simulink model "Test_PWM"  (R2014a)
settings: Solver=FixedStepDiscrete  StartTime=0.0  StopTime=10.0  FixedStep=0.1  RelTol=1e-3
libraries: GPIO_Lib x2, STM32_Config_Lib x1, TIMERS_Lib x1
settings Model: Creator=jan  LastModifiedBy=jan
settings DataIOCC: LimitDataPoints=off
settings OptimizationCC: OptimizeModelRefInitCode=on  LifeSpan=1
settings HardwareCC: ProdLargestAtomicInteger=Integer  ProdLargestAtomicFloat=Float  ProdIntDivRoundTo=Zero  ProdEndianess=LittleEndian  ProdHWDeviceType=STMicroelectronics->STM32 32-bit Cortex-M
settings RTWCC: SystemTargetFile=stm32.tlc  TemplateMakefile=stm32.tmf  Description=stm32 (Embedded Target)  GenerateReport=on  ProcessScript=stm32_make_rtw_hook  Toolchain=Microsoft Visual C++ 2012 v11.0 | nmake (64-bit Windows)
settings CodeAppCC: IgnoreCustomStorageClasses=off  MaxIdLength=64  CustomSymbolStrType=$N$R$M  SimulinkBlockComments=off
settings STFCustomTargetCC: CodeReplacementLibrary=ARM CMSIS SIN COS  ParMdlRefBuildCompliant=on  ConcurrentExecutionCompliant=off  IncludeMdlTerminateFcn=off  GeneratePreprocessorConditionals=Use local settings  CombineOutputUpdateFcns=on  ERTCustomFileBanners=on  SupportContinuousTime=off  MATLABClassNameForMDSCustomization=Simulink.SoftwareTarget.ERTCustomization  GRTInterface=off  SystemTargetFile=stm32.tlc
settings ERTTargetCC: CodeReplacementLibrary=ARM CMSIS SIN COS  GenerateSampleERTMain=off  ParMdlRefBuildCompliant=on  IncludeMdlTerminateFcn=off  SupportNonInlinedSFcns=on  ERTSrcFileBannerTemplate=sourceFileTemplate.cgt  ERTHdrFileBannerTemplate=sourceFileTemplate.cgt  ERTDataSrcFileTemplate=sourceFileTemplate.cgt  ERTDataHdrFileTemplate=sourceFileTemplate.cgt  ERTCustomFileTemplate=customRoutineProcess.tlc

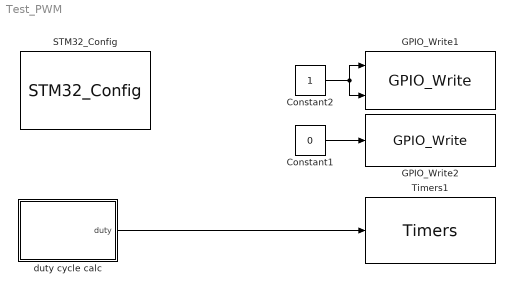
== system Test_PWM ==
  Constant1 : Constant  Value=0  OutDataTypeStr=uint8
  Constant2 : Constant  OutDataTypeStr=uint8
  GPIO_Write1 : GPIO_Lib/GPIO_Write  Port_name=GPIOC  Pin0=off  Toggle_Pin0=off  Pin1=off  Toggle_Pin1=off  Pin2=off  Toggle_Pin2=off  Pin3=off  Toggle_Pin3=off  Pin4=off  Toggle_Pin4=off  Pin5=off  Toggle_Pin5=off  Pin6=off  Toggle_Pin6=off  Pin7=off  Toggle_Pin7=off  Pin8=off  Toggle_Pin8=off  Pin9=off  Toggle_Pin9=off  Pin10=off  Toggle_Pin10=off  Pin11=off  Toggle_Pin11=off  Pin12=off  Toggle_Pin12=off  Pin13=on  Toggle_Pin13=off  Pin14=on  Toggle_Pin14=off  Pin15=off  Toggle_Pin15=off  PinList="GPIOA7GPIOC4   5  11  13  14GPIOD0   1   7  11  12  13  14  15GPIOE1  3  4"
  GPIO_Write2 : GPIO_Lib/GPIO_Write  Port_name=GPIOD  Pin0=off  Toggle_Pin0=off  Pin1=off  Toggle_Pin1=off  Pin2=off  Toggle_Pin2=off  Pin3=off  Toggle_Pin3=off  Pin4=off  Toggle_Pin4=off  Pin5=off  Toggle_Pin5=off  Pin6=off  Toggle_Pin6=off  Pin7=on  Toggle_Pin7=off  Pin8=off  Toggle_Pin8=off  Pin9=off  Toggle_Pin9=off  Pin10=off  Toggle_Pin10=off  Pin11=off  Toggle_Pin11=off  Pin12=off  Toggle_Pin12=off  Pin13=off  Toggle_Pin13=off  Pin14=off  Toggle_Pin14=off  Pin15=off  Toggle_Pin15=off  PinList="GPIOA7GPIOC4   5  11  13  14GPIOD0   1   7  11  12  13  14  15GPIOE1  3  4"
  STM32_Config : STM32_Config_Lib/STM32_Config  Priority=0  Project_Path=E:\HTWAA_car_32b\projects\Test_PWM\  Config_File=HTWAA_32b.ioc  MCU_Name=STM32F429VITx
  Timers1 : TIMERS_Lib/Timers  currentTIM=TIM9  TIM_Name=TIM9  TIM_APBClock=168000000  TIM_CKD=1  TIM_Set_Clk=off  TIM_Prescaler=0  TIM_Clock=168000000.00  Variable_frequency=off  TIM_Set_OutFreq=on  TIM_ARR=168000  Output_frequency=1000.00  Repetition_counter=0  TIM_Mode=Up  TIM_DMA=none  TIM_IRQ=off  TIM_UP=off  TIM_TRG=off  TIM_COM=off  TIM_BRK=off  NbTIM=6  CH1_enable=on  CH1N_enable=off  CH1_type=Output_PWM  CH1_DMA=off  CH1_int=off  CH1_edge=Rising  CH1_div=1  CH1_variable_duty=on  CH1_set_pulse=off  CH1_output_duty=0.00  CH1_pulse=0  CH2_enable=off  CH2N_enable=off  CH2_type=Unknown  CH2_DMA=off  CH2_int=off  CH2_edge=Rising  CH2_div=1  CH2_variable_duty=off  CH2_set_pulse=off  CH2_output_duty=0.00  CH2_pulse=0  CH3_enable=off  CH3N_enable=off  CH3_type=Unknown  CH3_DMA=off  CH3_int=off  CH3_edge=Rising  CH3_div=1  CH3_variable_duty=off  CH3_set_pulse=off  CH3_output_duty=0.00  CH3_pulse=0  CH4_enable=off  CH4N_enable=off  CH4_type=Unknown  CH4_DMA=off  CH4_int=off  CH4_edge=Rising  CH4_div=1  CH4_variable_duty=off  CH4_set_pulse=off  CH4_output_duty=0.00  CH4_pulse=0
  duty cycle calc : Stateflow chart  TreatAsAtomicUnit=on
  wires:
  Constant2/1 -> GPIO_Write1/2, GPIO_Write1/1
  Constant1/1 -> GPIO_Write2/1
  duty cycle calc/1(duty) -> Timers1/1

== stateflow chart Test_PWM/duty cycle calc ==
  state S1
    du: duty = 5;
  state S3
    du: duty = 80;
  state S2
    du: duty = 20;
  (default) -> S1
  S3 -> S1 : after(1,sec)
  S1 -> S2 : after(1,sec)
  S2 -> S3 : after(1,sec)
  data: duty output
